simulink model "grading_system"  (R2021a)
settings: Solver=FixedStepDiscrete  StartTime=0.0  StopTime=10.0  RelTol=1e-3  EnableMultiTasking=on
settings Model: Creator=elkny  LastModifiedBy=elkny
settings DataIOCC: ReturnWorkspaceOutputs=off
settings OptimizationCC: DefaultParameterBehavior=Inlined  InlineInvariantSignals=on  EnableMemcpy=off  LifeSpan=1  EfficientTunableParamExpr=on
settings DebuggingCC: UnderspecifiedInitializationDetection=Classic  MergeDetectMultiDrivingBlocksExec=none  SFMachineParentedDataDiag=warning  ArithmeticOperatorsInVariantConditions=warning
settings ModelReferenceCC: PropagateSignalLabelsOutOfModel=off
settings SFSimCC: MATLABDynamicMemAlloc=off  CustomCodeUndefinedFunction=UseInterfaceOnly
settings RTWCC: SystemTargetFile=ert.tlc  GenCodeOnly=on  TemplateMakefile=ert_default_tmf  GenerateReport=on  IncludeHyperlinkInReport=on  LaunchReport=on  GenerateTraceInfo=on  GenerateTraceReport=on  GenerateTraceReportSl=on  GenerateTraceReportSf=on  GenerateTraceReportEml=on
settings CodeAppCC: ForceParamTrailComments=on  IgnoreCustomStorageClasses=off  OperatorAnnotations=on  SimulinkDataObjDesc=on  SFDataObjDesc=on  MATLABFcnDesc=on  InsertBlockDesc=on  StateflowObjectComments=on  MATLABSourceComments=on
settings ERTTargetCC: MultiwordLength=2048  GenerateSampleERTMain=on  InlinedParameterPlacement=NonHierarchical  ERTCustomFileTemplate=example_file_process.tlc

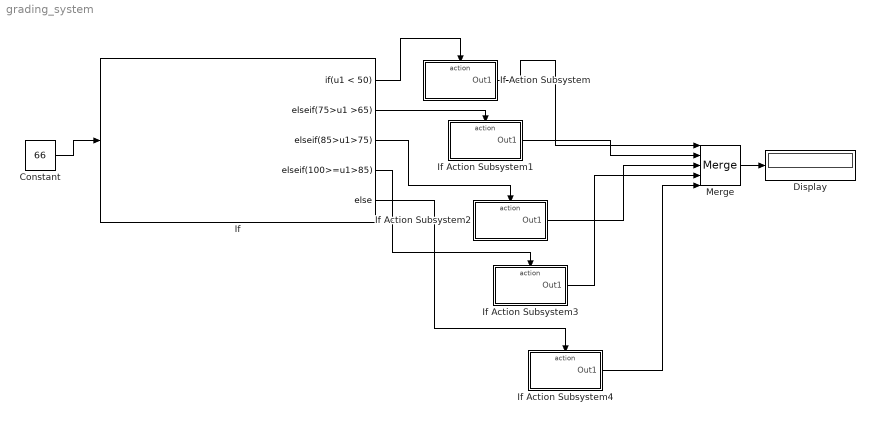
== system grading_system ==
  Constant : Constant  Value=66
  Display : Display
  If : If  IfExpression=u1 < 50  ElseIfExpressions="75>u1 >65 , 85>u1>75  , 100>=u1>85"
  If Action Subsystem : Subsystem  TreatAsAtomicUnit=on
  If Action Subsystem1 : Subsystem  TreatAsAtomicUnit=on
  If Action Subsystem2 : Subsystem  TreatAsAtomicUnit=on
  If Action Subsystem3 : Subsystem  TreatAsAtomicUnit=on
  If Action Subsystem4 : Subsystem  TreatAsAtomicUnit=on
  Merge : Merge  Inputs=5
  wires:
  If/1 -> If Action Subsystem/Action
  If Action Subsystem/1(Out1) -> Merge/1
  If/2 -> If Action Subsystem1/Action
  If/3 -> If Action Subsystem2/Action
  If/4 -> If Action Subsystem3/Action
  If/5 -> If Action Subsystem4/Action
  If Action Subsystem1/1(Out1) -> Merge/2
  If Action Subsystem2/1(Out1) -> Merge/3
  If Action Subsystem3/1(Out1) -> Merge/4
  If Action Subsystem4/1(Out1) -> Merge/5
  Merge/1 -> Display/1
  Constant/1 -> If/1

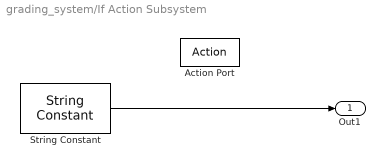
== system grading_system/If Action Subsystem ==
  Action Port : ActionPort  ActionPortLabel=if(u1 < 50)
  String Constant : StringConstant  String="\"failed\""
  Out1 : Outport
  wires:
  String Constant/1 -> Out1/1

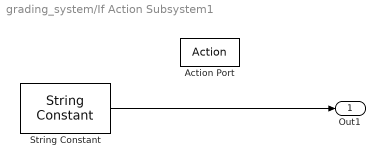
== system grading_system/If Action Subsystem1 ==
  Action Port : ActionPort  ActionPortLabel=elseif( 75>u1 >65 )
  String Constant : StringConstant  String="\"good\""
  Out1 : Outport
  wires:
  String Constant/1 -> Out1/1

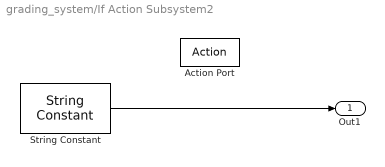
== system grading_system/If Action Subsystem2 ==
  Action Port : ActionPort  ActionPortLabel="elseif( 85>u1>75  )"
  String Constant : StringConstant  String="\"very good\""
  Out1 : Outport
  wires:
  String Constant/1 -> Out1/1

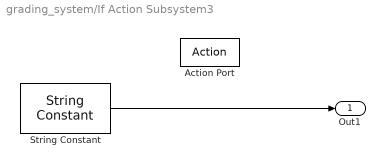
== system grading_system/If Action Subsystem3 ==
  Action Port : ActionPort  ActionPortLabel=elseif( 100>=u1>85)
  String Constant : StringConstant  String="\"excelent\""
  Out1 : Outport
  wires:
  String Constant/1 -> Out1/1

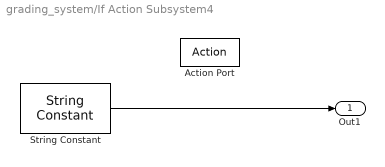
== system grading_system/If Action Subsystem4 ==
  Action Port : ActionPort  ActionPortLabel=else
  String Constant : StringConstant  String="\"invalid\""
  Out1 : Outport
  wires:
  String Constant/1 -> Out1/1
